simulink model "model"  (R2020a)
settings: Solver=VariableStepAuto  StartTime=0.0  StopTime=10.0  RelTol=1e-3
PreLoadFcn:
  | R=1/10
  | C=1/10*10^-6
  | a=1
  | for i=1:5
  |     a=a*2*10^-3;
  |     q=a;
  |     sim("Problem_5.slx",10);
  | end
settings Model: Creator=Avengers  LastModifiedBy=Avengers

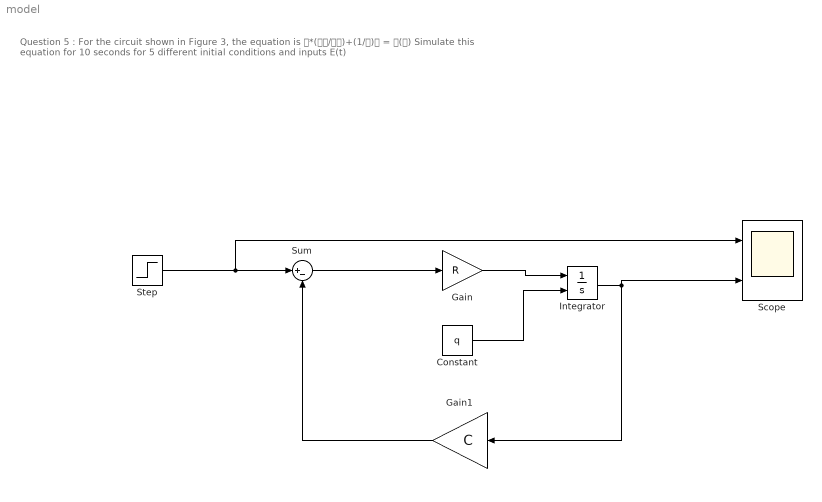
== system model ==
  note: Question 5 :
      | For the circuit shown in Figure 3, the equation is
      | 𝑅*(𝑑𝑄/𝑑𝑡)+(1/𝐶)𝑄 = 𝐸(𝑡)
      | Simulate this equation for 10 seconds for 5 different initial conditions and inputs E(t)
  Constant : Constant  Value=q
  Gain : Gain  Gain=R
  Gain1 : Gain  Gain=C
  Integrator : Integrator  InitialConditionSource=external
  Scope : Scope  NumInputPorts=2
  Step : Step  SampleTime=0
  Sum : Sum  Inputs=|+-
  wires:
  Integrator/1 -> Scope/2, Gain1/1
  Sum/1 -> Gain/1
  Gain1/1 -> Sum/2
  Constant/1 -> Integrator/2
  Gain/1 -> Integrator/1
  Step/1 -> Sum/1, Scope/1
